simulink model "disturbance_estimator"  (R2023b)
settings: Solver=VariableStepAuto  StartTime=0.0  StopTime=T  RelTol=1e-6
values from neighbouring files (symbols this model uses):
  k = coeff(r)    [main.m]
  r = input('Insert the order of the estimation: ')    [main.m]
  Ts = 0.001    [main.m]
settings Model: Creator=domen  LastModifiedBy=domen
settings OptimizationCC: ReuseModelBlockBuffer=off

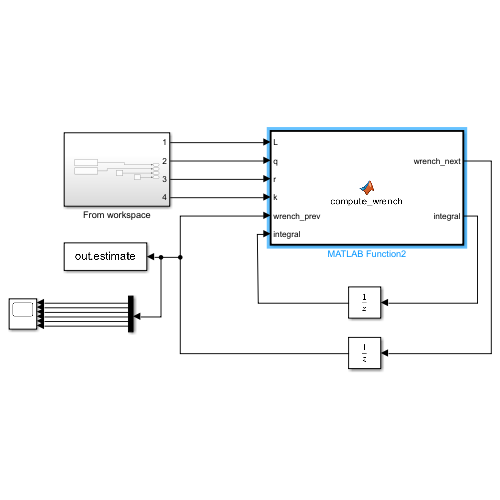
[thumbnail: Simulink's stored preview of the top-level diagram]
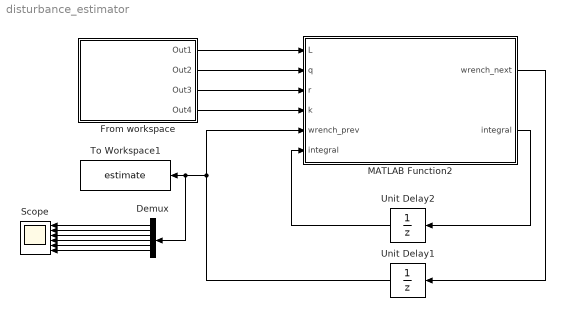
== system disturbance_estimator ==
  Demux : Demux  Outputs=6
  From workspace : Subsystem
  MATLAB Function2 : MATLAB Function  TreatAsAtomicUnit=on
  Scope : Scope  NumInputPorts=6
  To Workspace1 : ToWorkspace  VariableName=estimate  SaveFormat=Timeseries  SampleTime=-1
  Unit Delay1 : UnitDelay  InitialCondition=zeros(6,1)  SampleTime=Ts  HasFrameUpgradeWarning=on
  Unit Delay2 : UnitDelay  InitialCondition=zeros(6,r)  SampleTime=Ts  HasFrameUpgradeWarning=on
  wires:
  Unit Delay2/1 -> MATLAB Function2/6("integral ")
  Unit Delay1/1 -> MATLAB Function2/5(wrench_prev), Demux/1, To Workspace1/1
  MATLAB Function2/2(integral) -> Unit Delay2/1
  MATLAB Function2/1(wrench_next) -> Unit Delay1/1
  From workspace/1(Out1) -> MATLAB Function2/1(L)
  From workspace/2(Out2) -> MATLAB Function2/2(q)
  From workspace/3(Out3) -> MATLAB Function2/3(r)
  From workspace/4(Out4) -> MATLAB Function2/4(k)
  Demux/1 -> Scope/1
  Demux/2 -> Scope/2
  Demux/4 -> Scope/4
  Demux/5 -> Scope/5
  Demux/6 -> Scope/6
  Demux/3 -> Scope/3

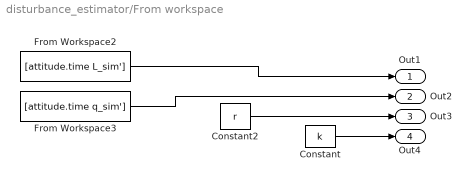
== system disturbance_estimator/From workspace ==
  Constant : Constant  Value=k
  Constant2 : Constant  Value=r
  From Workspace2 : FromWorkspace  VariableName=[attitude.time L_sim']  SampleTime=-1  OutputAfterFinalValue=Holding final value
  From Workspace3 : FromWorkspace  VariableName=[attitude.time q_sim']  SampleTime=-1  OutputAfterFinalValue=Holding final value
  Out1 : Outport
  Out2 : Outport  Port=2
  Out3 : Outport  Port=3
  Out4 : Outport  Port=4
  wires:
  Constant/1 -> Out4/1
  Constant2/1 -> Out3/1
  From Workspace3/1 -> Out2/1
  From Workspace2/1 -> Out1/1

== matlab function disturbance_estimator/MATLAB Function2 ==
  data: L input; q input; r input; k input; wrench_next output; wrench_prev input; integral output; integral input
function [wrench_next,integral] = compute_wrench(L,q,r,k,wrench_prev,integral)
    Ts=0.001;
    gamma=zeros(6,r);
    integral(:,1)=integral(:,1)+(wrench_prev+L)*Ts;
    gamma(:,1)=k(1)*(q-integral(:,1));
    for i=2:r 
        integral(:,i)=integral(:,i)+(-wrench_prev+gamma(:,i-1))*Ts;
        gamma(:,i)=k(i)*integral(:,i);   
    end
    wrench_next=gamma(:,r);
